simulink model "equivalent"  (R2018a)
settings: Solver=VariableStepAuto  StartTime=0.0  StopTime=10.0  RelTol=1e-3
undefined symbols (not defined in the file): DiscIntNeverNeededParam, sigbuilder_block
libraries: simulink x479
(part 1 of 10)
settings Model: Creator=cyfuzz  LastModifiedBy=ishaf
settings CodeAppCC: StateflowObjectComments=on

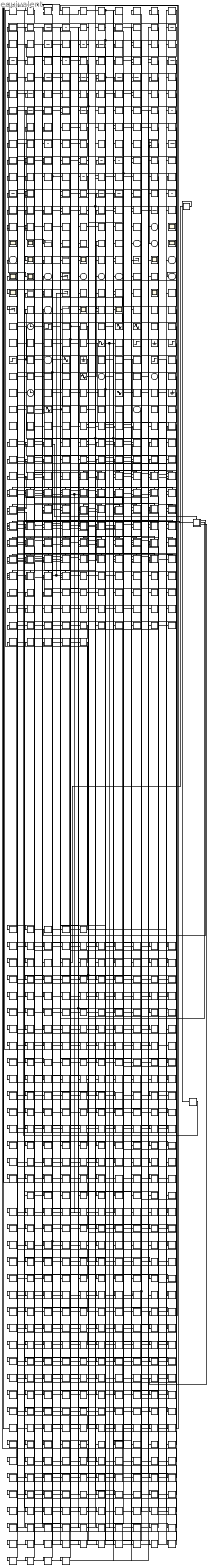
== system equivalent ==
  cfblk213 : Inport
  cfblk226 : Inport  Port=2
  cfblk229 : Inport  Port=3
  cfblk248 : Inport  Port=4
  cfblk{1,12,36,61,86,91,101,108,110,138} (10 alike) : simulink/Discrete/Transfer Fcn First Order  PoleZ=0.95  ICPrevOutput=0.0  DoSatur=off
      settings: SourceProductName=Simulink
  cfblk{10..11,16,21,37,63,66,76,80,123} (10 alike) : simulink/Continuous/PID Controller  Controller=PID  TimeDomain=Discrete-time  SampleTime=1  IntegratorMethod=Forward Euler  FilterMethod=Forward Euler  Form=Parallel  UseFilter=on  ControllerParametersSource=internal  P=1  I=1  D=0  N=100  InitialConditionSource=internal  InitialConditionForIntegrator=0  InitialConditionForFilter=0  ExternalReset=none  LimitOutput=off  UpperSaturationLimit=inf  LowerSaturationLimit=-inf  LinearizeAsGain=off  AntiWindupMode=none  Kb=1  TrackingMode=off  Kt=1  PParamMin=[]  PParamMax=[]  IParamMin=[]  IParamMax=[]  DParamMin=[]  DParamMax=[]  NParamMin=[]  NParamMax=[]  KbParamMin=[]  KbParamMax=[]  KtParamMin=[]  KtParamMax=[]  POutMin=[]  POutMax=[]  IOutMin=[]  IOutMax=[]  DOutMin=[]  DOutMax=[]  NOutMin=[]  NOutMax=[]  KbOutMin=[]  KbOutMax=[]  KtOutMin=[]  KtOutMax=[]  IntegratorOutMin=[]  IntegratorOutMax=[]  FilterOutMin=[]  FilterOutMax=[]  SumOutMin=[]  SumOutMax=[]  SumI1OutMin=[]  SumI1OutMax=[]  SumI2OutMin=[]  SumI2OutMax=[]  SumI3OutMin=[]  SumI3OutMax=[]  SumDOutMin=[]  SumDOutMax=[]  SaturationOutMin=[]  SaturationOutMax=[]  IntegratorContinuousStateAttributes=''  IntegratorStateMustResolveToSignalObject=off  IntegratorRTWStateStorageClass=Auto  FilterContinuousStateAttributes=''  FilterStateMustResolveToSignalObject=off  FilterRTWStateStorageClass=Auto  DifferentiatorICPrevScaledInput=0  DifferentiatorOutMin=[]  DifferentiatorOutMax=[]  FilterDiffOutCoefMin=[]  FilterDiffOutCoefMax=[]  SumDenOutMin=[]  SumDenOutMax=[]  SumNumOutMin=[]  SumNumOutMax=[]  ReciprocalOutMin=[]  ReciprocalOutMax=[]  DivideOutMin=[]  DivideOutMax=[]  TunerSelectOption=Transfer Function Based (PID Tuner App)
  cfblk{19,32,55,67,82,99..100,102,104,134} (10 alike) : simulink/Discrete/Difference  ICPrevInput=0.0  OutMin=[]  OutMax=[]  OutDataTypeStr=Inherit: Inherit via back propagation  OutDataType=fixdt(1, 16)  OutScaling=2^-10  DoSatur=off
  cfblk{33,42,49,57,103,121..122,126,135,345..384} (49 alike) : Delay  SampleTime=1
  cfblk{20,25,31,96,105,111} (6 alike) : DiscreteIntegrator  ICPrevOutput=DiscIntNeverNeededParam  ICPrevScaledInput=DiscIntNeverNeededParam
  cfblk{28,46,51,58,89,98,106,128} (8 alike) : simulink/Continuous/PID Controller (2DOF)  Controller=PID  TimeDomain=Discrete-time  SampleTime=1  IntegratorMethod=Forward Euler  FilterMethod=Forward Euler  Form=Parallel  UseFilter=on  ControllerParametersSource=internal  P=1  I=1  D=0  N=100  b=1  c=1  InitialConditionSource=internal  InitialConditionForIntegrator=0  InitialConditionForFilter=0  ExternalReset=none  LimitOutput=off  UpperSaturationLimit=inf  LowerSaturationLimit=-inf  LinearizeAsGain=off  AntiWindupMode=none  Kb=1  TrackingMode=off  Kt=1  PParamMin=[]  PParamMax=[]  IParamMin=[]  IParamMax=[]  DParamMin=[]  DParamMax=[]  NParamMin=[]  NParamMax=[]  bParamMin=[]  bParamMax=[]  cParamMin=[]  cParamMax=[]  KbParamMin=[]  KbParamMax=[]  KtParamMin=[]  KtParamMax=[]  POutMin=[]  POutMax=[]  IOutMin=[]  IOutMax=[]  DOutMin=[]  DOutMax=[]  NOutMin=[]  NOutMax=[]  bOutMin=[]  bOutMax=[]  cOutMin=[]  cOutMax=[]  KbOutMin=[]  KbOutMax=[]  KtOutMin=[]  KtOutMax=[]  IntegratorOutMin=[]  IntegratorOutMax=[]  FilterOutMin=[]  FilterOutMax=[]  SumOutMin=[]  SumOutMax=[]  Sum1OutMin=[]  Sum1OutMax=[]  Sum2OutMin=[]  Sum2OutMax=[]  Sum3OutMin=[]  Sum3OutMax=[]  SumI1OutMin=[]  SumI1OutMax=[]  SumI2OutMin=[]  SumI2OutMax=[]  SumI3OutMin=[]  SumI3OutMax=[]  SumDOutMin=[]  SumDOutMax=[]  SaturationOutMin=[]  SaturationOutMax=[]  IntegratorContinuousStateAttributes=''  IntegratorStateMustResolveToSignalObject=off  IntegratorRTWStateStorageClass=Auto  FilterContinuousStateAttributes=''  FilterStateMustResolveToSignalObject=off  FilterRTWStateStorageClass=Auto  DifferentiatorICPrevScaledInput=0  DifferentiatorOutMin=[]  DifferentiatorOutMax=[]  FilterDiffOutCoefMin=[]  FilterDiffOutCoefMax=[]  SumDenOutMin=[]  SumDenOutMax=[]  SumNumOutMin=[]  SumNumOutMax=[]  ReciprocalOutMin=[]  ReciprocalOutMax=[]  DivideOutMin=[]  DivideOutMax=[]  TunerSelectOption=Transfer Function Based (PID Tuner App)
  cfblk{35,53,87,94,107,119,125,133} (8 alike) : simulink/Discrete/Transfer Fcn Real Zero  ZeroZ=0.75  ICPrevInput=0.0  DoSatur=off
      settings: SourceProductName=Simulink  SourceProductBaseCode=SL
  cfblk{18,24,54,56,69,71,75,85,109,130} (10 alike) : simulink/Discrete/Transfer Fcn Lead or Lag  PoleZ=0.95  ZeroZ=0.75  ICPrevOutput=0.0  ICPrevInput=0.0  DoSatur=off
      settings: SourceProductName=Simulink  SourceProductBaseCode=SL
  cfblk{64,92,112,131..132} (5 alike) : Delay  DelayLengthSource=Input port  SampleTime=1
      settings: InputPortMap=u0,p1
  cfblk{7,15,22,27,30,41,44,60,81,113} (10 alike) : DiscreteZeroPole  Poles=[0 0.5]  Gain=1
  cfblk{3,38..39,77,93,95,114,124,127} (9 alike) : Delay  ShowEnablePort=on  SampleTime=1
      settings: InputPortMap=u0,e6
  cfblk{17,50,72,78..79,115} (6 alike) : simulink/Discrete/Tapped Delay  vinit=0.0  samptime=-1  NumDelays=1  DelayOrder=Oldest  includeCurrent=off
  cfblk{23,45,116..117} (4 alike) : DiscreteTransferFcn  SampleTime=1
  cfblk{2,4..6,59,68,73..74,118,137} (10 alike) : DiscreteFir  SampleTime=1
  cfblk{14,29,34,70,83,97,120} (7 alike) : UnitDelay
  cfblk{13,26,40,43,47..48,52,62,65,90,129} (11 alike) : DiscreteFilter  SampleTime=1
  cfblk{8..9,84,88,136} (5 alike) : DiscreteStateSpace
  cfblk{140..142,150,152,155,159,161..162,171,179,185,187} (13 alike) : Scope
      cfblk140 settings: Floating=on
      cfblk141 settings: Floating=on
      cfblk142 settings: Floating=on
      cfblk150 settings: Floating=on
      cfblk179 settings: Floating=on
  cfblk{143,154,172,184} (4 alike) : Display
  cfblk144 : ToWorkspace  VariableName=lgebsck  SaveFormat=Timeseries  SampleTime=-1
  cfblk145 : ToWorkspace  VariableName=bihdjlv  SaveFormat=Timeseries  SampleTime=-1
  cfblk{146,157,173,177,186} (5 alike) : simulink/Sinks/XY Graph  xmin=-1  xmax=1  ymin=-1  ymax=1  st=-1
  cfblk147 : ToWorkspace  VariableName=xeqpvpt  SaveFormat=Timeseries  SampleTime=-1
  cfblk153 : ToFile  Filename=ktyo  SaveFormat=Timeseries
  cfblk156 : ToFile  Filename=grzb  SaveFormat=Timeseries
  cfblk{158,164,174,181} (4 alike) : Terminator
  cfblk168 : ToWorkspace  VariableName=rlyvhgw  SaveFormat=Timeseries  SampleTime=-1
  cfblk169 : ToFile  Filename=ghct  SaveFormat=Timeseries
  cfblk175 : ToFile  Filename=zzva  SaveFormat=Timeseries
  cfblk176 : ToWorkspace  VariableName=iqauudf  SaveFormat=Timeseries  SampleTime=-1
  cfblk178 : ToFile  Filename=xfod  SaveFormat=Timeseries
  cfblk180 : ToWorkspace  VariableName=neyrlfn  SaveFormat=Timeseries  SampleTime=-1
  cfblk182 : ToFile  Filename=fvos  SaveFormat=Timeseries
  cfblk188 : ToWorkspace  VariableName=xtilwmv  SaveFormat=Timeseries  SampleTime=-1
  cfblk{189,203,231,247,250..251} (6 alike) : simulink/Sources/Repeating Sequence Interpolated  OutValues=[3 1 4 2 1].'  TimeValues=[0 0.1 0.5 0.6 1].'  LookUpMeth=Interpolation-Use End Values  tsamp=0.01  OutMin=[]  OutMax=[]  OutDataTypeStr=double  OutputDataTypeScalingMode=double  OutDataType=fixdt(0,8)  OutScaling=2^-10
  cfblk190 : simulink/Sources/Repeating Sequence  rep_seq_t=[0 2]  rep_seq_y=[0 2]
  cfblk191 : simulink/Sources/Repeating Sequence  rep_seq_t=[0 2]  rep_seq_y=[0 2]
  cfblk192 : Clock
  cfblk193 : Step  After=18  SampleTime=0
  cfblk194 : SignalGenerator  Units=rad/sec
  cfblk{195,216,234,236,238..239} (6 alike) : simulink/Sources/Chirp Signal  f1=0.1  T=100  f2=1
  cfblk196 : Constant  Value=8987
  cfblk{197..198,206,214,225,237,243} (7 alike) : Sin  SampleTime=0
  cfblk{199,230,235,241} (4 alike) : RandomNumber  SampleTime=0.1
  cfblk200 : simulink/Sources/Counter Free-Running  NumBits=16  tsamp=-1
  cfblk{201,212,220,249} (4 alike) : simulink/Sources/Band-Limited White Noise  Cov=[0.1]  Ts=0.1  seed=[23341]
  cfblk202 : UniformRandomNumber  SampleTime=0.1
  cfblk204 : Subsystem  Tag=STV Subsys  LoadFcn=sigbuilder_block('load');  StartFcn=sigbuilder_block('start');  StopFcn=sigbuilder_block('stop');  ClipboardFcn=sigbuilder_block('clipboard');  mask(Sigbuilder block){tuvar=[0:10]}
      mask help: Simulink:masks:SigbuilderBlock_MD
      mask init:
      | if ~strcmp(get_param(bdroot(gcbh),'SimulationStatus'),'stopped') tuvar = sigbuilder_block('maskInit'); end
      settings: CopyFcn=sigbuilder_block('copy');  DeleteFcn=sigbuilder_block('delete');  ModelCloseFcn=sigbuilder_block('modelClose');  PreSaveFcn=sigbuilder_block('preSave');  PauseFcn=sigbuilder_block('pause');  ContinueFcn=sigbuilder_block('continue');  NameChangeFcn=sigbuilder_block('namechange');  OpenFcn=sigbuilder_block('open',[437.6 199.2 550.4 400 ]);  CloseFcn=sigbuilder_block('close');
      mask Display: plot(0, 0, 100, 100,[2, 2, 32, 32, 2], [68, 8, 8, 68, 68],[32, 2], [38, 38], [32, 19, 2],[53, 60, 44], [32, 17, 17, 2],[16, 16, 31, 31]);txt = getActiveGroup(gcbh);text(2, 100, txt,'verticalAlignment', 'top');
  cfblk205 : DiscretePulseGenerator  PulseType=Time based  Period=10  PulseWidth=5
  cfblk207 : simulink/Sources/Repeating Sequence  rep_seq_t=[0 2]  rep_seq_y=[0 2]
  cfblk208 : Step  After=83  SampleTime=0
  cfblk209 : Ground
  cfblk210 : Step  After=27  SampleTime=0
  cfblk211 : Step  After=11  SampleTime=0
  cfblk215 : Ground
  cfblk{217,222,253..254} (4 alike) : simulink/Sources/Repeating Sequence Stair  OutValues=[3 1 4 2 1].'  tsamp=-1  OutMin=[]  OutMax=[]  OutDataTypeStr=double  OutputDataTypeScalingMode=double  OutDataType=fixdt(0,8)  ConRadixGroup=Best Precision: Vector-wise  OutScaling=2^-12
  cfblk218 : Constant  Value=1094
  cfblk219 : Step  After=49  SampleTime=0
  cfblk221 : DigitalClock
  cfblk223 : simulink/Sources/Ramp  slope=1  start=0  InitialOutput=0
  cfblk224 : Constant  Value=9975
  cfblk227 : simulink/Sources/Counter Limited  uplimit=7  tsamp=-1
  cfblk228 : Subsystem  Tag=STV Subsys  LoadFcn=sigbuilder_block('load');  StartFcn=sigbuilder_block('start');  StopFcn=sigbuilder_block('stop');  ClipboardFcn=sigbuilder_block('clipboard');  mask(Sigbuilder block){tuvar=[0:10]}
      mask help: Simulink:masks:SigbuilderBlock_MD
      mask init:
      | if ~strcmp(get_param(bdroot(gcbh),'SimulationStatus'),'stopped') tuvar = sigbuilder_block('maskInit'); end
      settings: CopyFcn=sigbuilder_block('copy');  DeleteFcn=sigbuilder_block('delete');  ModelCloseFcn=sigbuilder_block('modelClose');  PreSaveFcn=sigbuilder_block('preSave');  PauseFcn=sigbuilder_block('pause');  ContinueFcn=sigbuilder_block('continue');  NameChangeFcn=sigbuilder_block('namechange');  OpenFcn=sigbuilder_block('open',[437.6 199.2 550.4 400 ]);  CloseFcn=sigbuilder_block('close');
      mask Display: plot(0, 0, 100, 100,[2, 2, 32, 32, 2], [68, 8, 8, 68, 68],[32, 2], [38, 38], [32, 19, 2],[53, 60, 44], [32, 17, 17, 2],[16, 16, 31, 31]);txt = getActiveGroup(gcbh);text(2, 100, txt,'verticalAlignment', 'top');
  cfblk232 : Clock
  cfblk233 : SignalGenerator  Units=rad/sec
  cfblk240 : Ground
  cfblk242 : Subsystem  Tag=STV Subsys  LoadFcn=sigbuilder_block('load');  StartFcn=sigbuilder_block('start');  StopFcn=sigbuilder_block('stop');  ClipboardFcn=sigbuilder_block('clipboard');  mask(Sigbuilder block){tuvar=[0:10]}
      mask help: Simulink:masks:SigbuilderBlock_MD
      mask init:
      | if ~strcmp(get_param(bdroot(gcbh),'SimulationStatus'),'stopped') tuvar = sigbuilder_block('maskInit'); end
      settings: CopyFcn=sigbuilder_block('copy');  DeleteFcn=sigbuilder_block('delete');  ModelCloseFcn=sigbuilder_block('modelClose');  PreSaveFcn=sigbuilder_block('preSave');  PauseFcn=sigbuilder_block('pause');  ContinueFcn=sigbuilder_block('continue');  NameChangeFcn=sigbuilder_block('namechange');  OpenFcn=sigbuilder_block('open',[437.6 199.2 550.4 400 ]);  CloseFcn=sigbuilder_block('close');
      mask Display: plot(0, 0, 100, 100,[2, 2, 32, 32, 2], [68, 8, 8, 68, 68],[32, 2], [38, 38], [32, 19, 2],[53, 60, 44], [32, 17, 17, 2],[16, 16, 31, 31]);txt = getActiveGroup(gcbh);text(2, 100, txt,'verticalAlignment', 'top');
  cfblk244 : simulink/Sources/Counter Limited  uplimit=7  tsamp=-1
  cfblk245 : SignalGenerator  Units=rad/sec
  cfblk246 : DigitalClock
  cfblk252 : DigitalClock
  cfblk{255..284} (30 alike) : If  SampleTime=1
  cfblk285 : Subsystem  TreatAsAtomicUnit=on
  cfblk286 : Subsystem  TreatAsAtomicUnit=on
  cfblk287 : Subsystem  TreatAsAtomicUnit=on
  cfblk288 : Subsystem  TreatAsAtomicUnit=on
  cfblk289 : Subsystem  TreatAsAtomicUnit=on
  cfblk290 : Subsystem  TreatAsAtomicUnit=on
  cfblk291 : Subsystem  TreatAsAtomicUnit=on
  cfblk292 : Subsystem  TreatAsAtomicUnit=on
  cfblk293 : Subsystem  TreatAsAtomicUnit=on
  cfblk294 : Subsystem  TreatAsAtomicUnit=on
  cfblk295 : Subsystem  TreatAsAtomicUnit=on
  cfblk296 : Subsystem  TreatAsAtomicUnit=on
  cfblk297 : Subsystem  TreatAsAtomicUnit=on
  cfblk298 : Subsystem  TreatAsAtomicUnit=on
  cfblk299 : Subsystem  TreatAsAtomicUnit=on
  cfblk300 : Subsystem  TreatAsAtomicUnit=on
  cfblk301 : Subsystem  TreatAsAtomicUnit=on
  cfblk302 : Subsystem  TreatAsAtomicUnit=on
  cfblk303 : Subsystem  TreatAsAtomicUnit=on
  cfblk304 : Subsystem  TreatAsAtomicUnit=on
  cfblk305 : Subsystem  TreatAsAtomicUnit=on
  cfblk306 : Subsystem  TreatAsAtomicUnit=on
  cfblk307 : Subsystem  TreatAsAtomicUnit=on
  cfblk308 : Subsystem  TreatAsAtomicUnit=on
  cfblk309 : Subsystem  TreatAsAtomicUnit=on
  cfblk310 : Subsystem  TreatAsAtomicUnit=on
  cfblk311 : Subsystem  TreatAsAtomicUnit=on
  cfblk312 : Subsystem  TreatAsAtomicUnit=on
  cfblk313 : Subsystem  TreatAsAtomicUnit=on
  cfblk314 : Subsystem  TreatAsAtomicUnit=on
  cfblk315 : Subsystem  TreatAsAtomicUnit=on
  cfblk316 : Subsystem  TreatAsAtomicUnit=on
  cfblk317 : Subsystem  TreatAsAtomicUnit=on
  cfblk318 : Subsystem  TreatAsAtomicUnit=on
  cfblk319 : Subsystem  TreatAsAtomicUnit=on
  cfblk320 : Subsystem  TreatAsAtomicUnit=on
  cfblk321 : Subsystem  TreatAsAtomicUnit=on
  cfblk322 : Subsystem  TreatAsAtomicUnit=on
  cfblk323 : Subsystem  TreatAsAtomicUnit=on
  cfblk324 : Subsystem  TreatAsAtomicUnit=on
  cfblk325 : Subsystem  TreatAsAtomicUnit=on
  cfblk326 : Subsystem  TreatAsAtomicUnit=on
  cfblk327 : Subsystem  TreatAsAtomicUnit=on
  cfblk328 : Subsystem  TreatAsAtomicUnit=on
  cfblk329 : Subsystem  TreatAsAtomicUnit=on
  cfblk330 : Subsystem  TreatAsAtomicUnit=on
  cfblk331 : Subsystem  TreatAsAtomicUnit=on
  cfblk332 : Subsystem  TreatAsAtomicUnit=on
  cfblk333 : Subsystem  TreatAsAtomicUnit=on
  cfblk334 : Subsystem  TreatAsAtomicUnit=on
  cfblk335 : Subsystem  TreatAsAtomicUnit=on
  cfblk336 : Subsystem  TreatAsAtomicUnit=on
  cfblk337 : Subsystem  TreatAsAtomicUnit=on
  cfblk338 : Subsystem  TreatAsAtomicUnit=on
  cfblk339 : Subsystem  TreatAsAtomicUnit=on
  cfblk340 : Subsystem  TreatAsAtomicUnit=on
  cfblk341 : Subsystem  TreatAsAtomicUnit=on
  cfblk342 : Subsystem  TreatAsAtomicUnit=on
  cfblk343 : Subsystem  TreatAsAtomicUnit=on
  cfblk344 : Subsystem  TreatAsAtomicUnit=on
  cfblk385 : DataTypeConversion  OutDataTypeStr=double
  cyemi_{0..42,44..47,49..57,59..77,79..113,124,165..166,202..203,210..211,215..218,228..229,234..236,304..306,349..351,361..362,372..373,447..448,450..451,457..459,498..502,517..518,557,595..596,634..635,663..667,705,723..728,739..740,773..774,789..791,805..808,816..817,827..828,889,929..932,955..956,963,970..971,987..988,1002..1004,1061..1062,1088..1089,1103..1104,1155..1157,1230..1231,1236..1240,1246..1247,1282..1284,1291..1292,1302..1303,1376..1377,1414..1415,1423..1424,1448..1449,1470,1538,1546..1548,1560..1562,1567..1568,1604..1605,1639..1641,1683,1692,1708..1710,1747..1791,1793..1859,1861..1870} (372 alike) : DataTypeConversion  OutDataTypeStr=double
  cyemi_1792 : DataTypeConversion  OutDataTypeStr=uint16
  cyemi_{43,48,237,1860} (4 alike) : DataTypeConversion  OutDataTypeStr=uint32
  cyemi_58 : DataTypeConversion  OutDataTypeStr=uint8
  cyemi_78 : DataTypeConversion  OutDataTypeStr=uint8
  cfblk139 : Outport
  cfblk148 : Outport  Port=2
  cfblk149 : Outport  Port=3
  cfblk151 : Outport  Port=4
  cfblk160 : Outport  Port=5
  cfblk163 : Outport  Port=6
  cfblk165 : Outport  Port=7
  cfblk166 : Outport  Port=8
  cfblk167 : Outport  Port=9
  cfblk170 : Outport  Port=10
  cfblk183 : Outport  Port=11
  wires:
  cfblk79/1 -> cfblk149/1
  cfblk61/1 -> cfblk143/1
  cfblk2/1 -> cfblk162/1
  cfblk10/1 -> cfblk148/1
  cfblk225/1 -> cfblk146/1
  cfblk323/1(cfblk2) -> cfblk183/1
  cfblk46/1 -> cyemi_457/1, cyemi_1568/1
  cfblk197/1 -> cfblk172/1
  cfblk7/1 -> cfblk181/1
  cfblk307/1(cfblk2) -> cfblk166/1
  cfblk243/1 -> cyemi_727/1, cyemi_1846/1, cfblk177/2
  cfblk20/1 -> cyemi_110/1, cyemi_1548/1
  cfblk194/1 -> cyemi_38/1, cyemi_740/1
  cfblk206/1 -> cyemi_667/1, cyemi_1853/1
  cfblk217/1 -> cyemi_1088/1, cyemi_1239/1
  cfblk8/1 -> cfblk186/1
  cfblk69/1 -> cyemi_29/1, cyemi_236/1
  cfblk211/1 -> cfblk146/2, cyemi_666/1
  cfblk214/1 -> cyemi_234/1, cyemi_1867/1
  cfblk314/2(cfblk8) -> cfblk160/1
  cfblk80/1 -> cfblk170/1
  cfblk118/1 -> cfblk186/2, cyemi_1778/1
  cfblk290/1(cfblk2) -> cfblk151/1
  cfblk231/1 -> cyemi_22/1, cyemi_932/1
  cfblk98/1 -> cyemi_235/1, cyemi_1753/1
  cfblk195/1 -> cyemi_1869/1, cyemi_1870/1
  cfblk301/1(cfblk2) -> cfblk139/1
  cfblk38/1 -> cyemi_1284/1, cyemi_1424/1
  cfblk298/2(cfblk9) -> cfblk159/1, cyemi_106/1
  cfblk343/1(cfblk2) -> cfblk174/1, cyemi_82/1
  cfblk310/4(cfblk16) -> cfblk161/1
  cfblk29/1 -> cfblk152/1
  cfblk330/2(cfblk13) -> cfblk165/1
  cfblk125/1 -> cfblk155/1
  cfblk335/2(cfblk11) -> cfblk157/1
  cfblk312/1(cfblk2) -> cyemi_725/1, cyemi_1758/1
  cfblk331/3(cfblk11) -> cfblk154/1
  cfblk103/1 -> cyemi_728/1, cyemi_1777/1
  cfblk57/1 -> cfblk158/1
  cfblk301/2(cfblk13) -> cfblk187/1
  cfblk34/1 -> cyemi_54/1, cyemi_1710/1
  cfblk81/1 -> cfblk157/2
  cfblk331/4(cfblk12) -> cfblk184/1
  cfblk21/1 -> cfblk167/1
  cfblk16/1 -> cyemi_889/1, cyemi_1546/1
  cfblk229/1 -> cyemi_237/1, cyemi_1860/1
  cfblk304/1(cfblk2) -> cfblk173/1
  cfblk18/1 -> cfblk164/1
  cfblk25/1 -> cfblk185/1
  cfblk294/2(cfblk14) -> cyemi_21/1, cyemi_726/1
  cfblk60/1 -> cyemi_1240/1, cyemi_1811/1
  cfblk295/2(cfblk11) -> cfblk173/2
  cfblk134/1 -> cfblk171/1
  cfblk6/1 -> cyemi_10/1, cyemi_963/1
  cfblk320/4(cfblk15) -> cfblk163/1
  cfblk106/1 -> cfblk177/1
  cfblk255/1 -> cfblk285/Action
  cfblk255/2 -> cfblk286/Action
  cfblk256/1 -> cfblk287/Action
  cfblk256/2 -> cfblk288/Action
  cfblk257/1 -> cfblk289/Action
  cfblk257/2 -> cfblk290/Action
  cfblk258/1 -> cfblk291/Action
  cfblk258/2 -> cfblk292/Action
  cfblk259/1 -> cfblk293/Action
  cfblk259/2 -> cfblk294/Action
  cfblk260/1 -> cfblk295/Action
  cfblk260/2 -> cfblk296/Action
  cfblk261/1 -> cfblk297/Action
  cfblk261/2 -> cfblk298/Action
  cfblk262/1 -> cfblk299/Action
  cfblk262/2 -> cfblk300/Action
  cfblk263/1 -> cfblk301/Action
  cfblk263/2 -> cfblk302/Action
  cfblk264/1 -> cfblk303/Action
  cfblk264/2 -> cfblk304/Action
  cfblk265/1 -> cfblk305/Action
  cfblk265/2 -> cfblk306/Action
  cfblk266/1 -> cfblk307/Action
  cfblk266/2 -> cfblk308/Action
  cfblk267/1 -> cfblk309/Action
  cfblk267/2 -> cfblk310/Action
  cfblk268/1 -> cfblk311/Action
  cfblk268/2 -> cfblk312/Action
  cfblk269/1 -> cfblk313/Action
  cfblk269/2 -> cfblk314/Action
  cfblk270/1 -> cfblk315/Action
  cfblk270/2 -> cfblk316/Action
  cfblk271/1 -> cfblk317/Action
  cfblk271/2 -> cfblk318/Action
  cfblk272/1 -> cfblk319/Action
  cfblk272/2 -> cfblk320/Action
  cfblk273/1 -> cfblk321/Action
  cfblk273/2 -> cfblk322/Action
  cfblk274/1 -> cfblk323/Action
  cfblk274/2 -> cfblk324/Action
  cfblk275/1 -> cfblk325/Action
  cfblk275/2 -> cfblk326/Action
  cfblk276/1 -> cfblk327/Action
  cfblk276/2 -> cfblk328/Action
  cfblk277/1 -> cfblk329/Action
  cfblk277/2 -> cfblk330/Action
  cfblk278/1 -> cfblk331/Action
  cfblk278/2 -> cfblk332/Action
  cfblk279/1 -> cfblk333/Action
  cfblk279/2 -> cfblk334/Action
  cfblk280/1 -> cfblk335/Action
  cfblk280/2 -> cfblk336/Action
  cfblk281/1 -> cfblk337/Action
  cfblk281/2 -> cfblk338/Action
  cfblk282/1 -> cfblk339/Action
  cfblk282/2 -> cfblk340/Action
  cfblk283/1 -> cfblk341/Action
  cfblk283/2 -> cfblk342/Action
  cfblk284/1 -> cfblk343/Action
  cfblk284/2 -> cfblk344/Action
  cyemi_0/1 -> cfblk1/1
  cfblk362/1 -> cyemi_0/1
  cyemi_1/1 -> cfblk10/1
  cfblk315/4(cfblk13) -> cyemi_1/1
  cyemi_2/1 -> cfblk100/1
  cfblk302/1(cfblk2) -> cyemi_2/1
  cyemi_3/1 -> cfblk101/1
  cfblk286/1(cfblk2) -> cyemi_3/1
  cyemi_4/1 -> cfblk102/1
  cfblk293/2(cfblk12) -> cyemi_4/1
  cyemi_5/1 -> cfblk103/1
  cfblk314/1(cfblk2) -> cyemi_5/1
  cyemi_6/1 -> cfblk104/1
  cfblk230/1 -> cyemi_6/1
  cyemi_7/1 -> cfblk105/1
  cfblk296/1(cfblk2) -> cyemi_7/1
  cyemi_8/1 -> cfblk106/1
  cfblk224/1 -> cyemi_8/1
  cyemi_9/1 -> cfblk106/2
  cfblk338/2(cfblk8) -> cyemi_9/1
  cyemi_10/1 -> cfblk107/1
  cyemi_11/1 -> cfblk108/1
  cfblk47/1 -> cyemi_11/1
  cyemi_12/1 -> cfblk109/1
  cfblk205/1 -> cyemi_12/1
  cyemi_13/1 -> cfblk11/1
  cfblk122/1 -> cyemi_13/1
  cyemi_14/1 -> cfblk110/1
  cfblk56/1 -> cyemi_14/1
  cyemi_15/1 -> cfblk111/1
  cfblk327/1(cfblk2) -> cyemi_15/1
  cyemi_16/1 -> cfblk112/1
  cfblk108/1 -> cyemi_16/1
  cyemi_17/1 -> cfblk112/2
  cfblk201/1 -> cyemi_17/1
  cyemi_18/1 -> cfblk113/1
  cfblk385/1 -> cyemi_18/1
  cyemi_19/1 -> cfblk114/1
  cfblk221/1 -> cyemi_19/1
  cyemi_20/1 -> cfblk114/2
  cfblk213/1 -> cyemi_20/1
  cyemi_21/1 -> cfblk115/1
  cyemi_22/1 -> cfblk116/1
  cyemi_23/1 -> cfblk117/1
  cfblk107/1 -> cyemi_23/1
  cyemi_24/1 -> cfblk118/1
  cfblk334/1(cfblk2) -> cyemi_24/1
  cyemi_25/1 -> cfblk119/1
  cfblk331/1(cfblk2) -> cyemi_25/1
  cyemi_26/1 -> cfblk12/1
  cfblk320/1(cfblk2) -> cyemi_26/1
  cyemi_27/1 -> cfblk120/1
  cfblk291/1(cfblk2) -> cyemi_27/1
  cyemi_28/1 -> cfblk121/1
  cfblk316/1(cfblk2) -> cyemi_28/1
  cyemi_29/1 -> cfblk122/1
  cyemi_30/1 -> cfblk123/1
  cfblk136/1 -> cyemi_30/1
  cyemi_31/1 -> cfblk124/1
  cfblk70/1 -> cyemi_31/1
  cyemi_32/1 -> cfblk124/2
  cfblk333/1(cfblk2) -> cyemi_32/1
  cyemi_33/1 -> cfblk125/1
  cfblk252/1 -> cyemi_33/1
  cyemi_34/1 -> cfblk126/1
  cfblk239/1 -> cyemi_34/1
  cyemi_35/1 -> cfblk127/1
  cfblk382/1 -> cyemi_35/1
  cyemi_36/1 -> cfblk127/2
  cfblk83/1 -> cyemi_36/1
  cyemi_37/1 -> cfblk128/1
  cfblk299/3(cfblk15) -> cyemi_37/1
  cyemi_38/1 -> cfblk128/2
  cyemi_39/1 -> cfblk129/1
  cfblk9/1 -> cyemi_39/1
  cyemi_40/1 -> cfblk13/1
  cfblk189/1 -> cyemi_40/1
  cyemi_41/1 -> cfblk130/1
  cfblk314/3(cfblk9) -> cyemi_41/1
  cyemi_42/1 -> cfblk131/1
  cfblk287/1(cfblk2) -> cyemi_42/1
  cyemi_43/1 -> cfblk131/2
  cfblk135/1 -> cyemi_43/1
  cyemi_44/1 -> cfblk132/1
  cfblk367/1 -> cyemi_44/1
  cyemi_45/1 -> cfblk132/2
  cfblk304/3(cfblk9) -> cyemi_45/1
  cyemi_46/1 -> cfblk133/1
  cfblk44/1 -> cyemi_46/1
  cyemi_47/1 -> cfblk134/1
  cfblk286/2(cfblk10) -> cyemi_47/1
  cyemi_48/1 -> cfblk135/1
  cfblk302/2(cfblk13) -> cyemi_48/1
  cyemi_49/1 -> cfblk136/1
  cfblk28/1 -> cyemi_49/1
  cyemi_50/1 -> cfblk137/1
  cfblk305/1(cfblk2) -> cyemi_50/1
  cyemi_51/1 -> cfblk138/1
  cfblk67/1 -> cyemi_51/1
  cyemi_52/1 -> cfblk14/1
  cfblk84/1 -> cyemi_52/1
  cyemi_53/1 -> cfblk144/1
  cfblk325/2(cfblk7) -> cyemi_53/1
  cyemi_54/1 -> cfblk145/1
  cyemi_55/1 -> cfblk147/1
  cfblk328/2(cfblk9) -> cyemi_55/1
  cyemi_56/1 -> cfblk15/1
  cfblk112/1 -> cyemi_56/1
  cyemi_57/1 -> cfblk153/1
  cfblk326/2(cfblk10) -> cyemi_57/1
  cyemi_58/1 -> cfblk156/1
  cfblk244/1 -> cyemi_58/1
  cyemi_59/1 -> cfblk16/1
  cfblk242/1(Signal 1) -> cyemi_59/1
  cyemi_60/1 -> cfblk168/1
  cfblk330/3(cfblk14) -> cyemi_60/1
  cyemi_61/1 -> cfblk169/1
  cfblk303/1(cfblk2) -> cyemi_61/1
  cyemi_62/1 -> cfblk17/1
  cfblk316/3(cfblk11) -> cyemi_62/1
  cyemi_63/1 -> cfblk175/1
  cfblk92/1 -> cyemi_63/1
  cyemi_64/1 -> cfblk176/1
  cfblk289/2(cfblk7) -> cyemi_64/1
  cyemi_65/1 -> cfblk178/1
  cfblk137/1 -> cyemi_65/1
  cyemi_66/1 -> cfblk18/1
  cfblk119/1 -> cyemi_66/1
  cyemi_67/1 -> cfblk180/1
  cfblk104/1 -> cyemi_67/1
  cyemi_68/1 -> cfblk182/1
  cfblk85/1 -> cyemi_68/1
  cyemi_69/1 -> cfblk188/1
  cfblk138/1 -> cyemi_69/1
  cyemi_70/1 -> cfblk19/1
  cfblk121/1 -> cyemi_70/1
  cyemi_71/1 -> cfblk2/1
  cfblk323/2(cfblk17) -> cyemi_71/1
  cyemi_72/1 -> cfblk20/1
  cfblk199/1 -> cyemi_72/1
  cyemi_73/1 -> cfblk21/1
  cfblk74/1 -> cyemi_73/1
  cyemi_74/1 -> cfblk22/1
  cfblk222/1 -> cyemi_74/1
  cyemi_75/1 -> cfblk23/1
  cfblk55/1 -> cyemi_75/1
  cyemi_76/1 -> cfblk24/1
  cfblk308/1(cfblk2) -> cyemi_76/1
  cyemi_77/1 -> cfblk25/1
  cfblk51/1 -> cyemi_77/1
  cyemi_78/1 -> cfblk255/1
  cfblk227/1 -> cyemi_78/1
  cyemi_79/1 -> cfblk256/1
  cfblk310/2(cfblk14) -> cyemi_79/1
  cyemi_80/1 -> cfblk257/1
  cfblk384/1 -> cyemi_80/1
  cyemi_81/1 -> cfblk258/1
  cfblk226/1 -> cyemi_81/1
  cyemi_82/1 -> cfblk259/1
  cyemi_83/1 -> cfblk26/1
  cfblk228/1(Signal 1) -> cyemi_83/1
  cyemi_84/1 -> cfblk260/1
  cfblk68/1 -> cyemi_84/1
  cyemi_85/1 -> cfblk261/1
  cfblk251/1 -> cyemi_85/1
  cyemi_86/1 -> cfblk262/1
  cfblk296/3(cfblk13) -> cyemi_86/1
  cyemi_87/1 -> cfblk263/1
  cfblk358/1 -> cyemi_87/1
  cyemi_88/1 -> cfblk264/1
  cfblk319/1(cfblk2) -> cyemi_88/1
  cyemi_89/1 -> cfblk265/1
  cfblk249/1 -> cyemi_89/1
  cyemi_90/1 -> cfblk266/1
  cfblk332/4(cfblk12) -> cyemi_90/1
  cyemi_91/1 -> cfblk267/1
  cfblk202/1 -> cyemi_91/1
  cyemi_92/1 -> cfblk268/1
  cfblk115/1 -> cyemi_92/1
  cyemi_93/1 -> cfblk269/1
  cfblk128/1 -> cyemi_93/1
  cyemi_94/1 -> cfblk27/1
  cfblk311/1(cfblk2) -> cyemi_94/1
  cyemi_95/1 -> cfblk270/1
  cfblk240/1 -> cyemi_95/1
  cyemi_96/1 -> cfblk271/1
  cfblk82/1 -> cyemi_96/1
  cyemi_97/1 -> cfblk272/1
  cfblk191/1 -> cyemi_97/1
  cyemi_98/1 -> cfblk273/1
  cfblk348/1 -> cyemi_98/1
  cyemi_99/1 -> cfblk274/1
  cfblk15/1 -> cyemi_99/1
  cyemi_100/1 -> cfblk275/1
  cfblk130/1 -> cyemi_100/1
  cyemi_101/1 -> cfblk276/1
  cfblk131/1 -> cyemi_101/1
  cyemi_102/1 -> cfblk277/1
  cfblk190/1 -> cyemi_102/1
  cyemi_103/1 -> cfblk278/1
  cfblk340/1(cfblk2) -> cyemi_103/1
  cyemi_104/1 -> cfblk279/1
  cfblk219/1 -> cyemi_104/1
  cyemi_105/1 -> cfblk28/1
  cfblk52/1 -> cyemi_105/1
  cyemi_106/1 -> cfblk28/2
  cyemi_107/1 -> cfblk280/1
  cfblk87/1 -> cyemi_107/1
  cyemi_108/1 -> cfblk281/1
  cfblk65/1 -> cyemi_108/1
  cyemi_109/1 -> cfblk282/1
  cfblk204/1(Signal 1) -> cyemi_109/1
  cyemi_110/1 -> cfblk283/1
  cyemi_111/1 -> cfblk284/1
  cfblk48/1 -> cyemi_111/1
  cyemi_112/1 -> cfblk285/1(cfblk1)
  cfblk99/1 -> cyemi_112/1
  cyemi_113/1 -> cfblk285/2(cfblk11)
  cfblk313/3(cfblk15) -> cyemi_113/1
  cyemi_124/1 -> cfblk286/1(cfblk1)
  cfblk114/1 -> cyemi_124/1
  cyemi_165/1 -> cfblk287/1(cfblk1)
  cfblk208/1 -> cyemi_165/1
  cyemi_166/1 -> cfblk287/2(cfblk12)
  cfblk340/2(cfblk13) -> cyemi_166/1
  cyemi_202/1 -> cfblk288/1(cfblk1)
  cfblk58/1 -> cyemi_202/1
  cyemi_203/1 -> cfblk288/2(cfblk7)
  cfblk310/3(cfblk15) -> cyemi_203/1
  cyemi_210/1 -> cfblk289/1(cfblk1)
  cfblk45/1 -> cyemi_210/1
  cyemi_211/1 -> cfblk289/2(cfblk6)
  cfblk245/1 -> cyemi_211/1
  cyemi_215/1 -> cfblk29/1
  cfblk31/1 -> cyemi_215/1
  cyemi_216/1 -> cfblk290/1(cfblk1)
  cfblk378/1 -> cyemi_216/1
  cyemi_217/1 -> cfblk290/2(cfblk9)
  cfblk346/1 -> cyemi_217/1
  cyemi_218/1 -> cfblk290/3(cfblk10)
  cfblk42/1 -> cyemi_218/1
  cyemi_228/1 -> cfblk291/1(cfblk1)
  cfblk342/1(cfblk2) -> cyemi_228/1
  cyemi_229/1 -> cfblk291/2(cfblk7)
  cfblk27/1 -> cyemi_229/1
  cyemi_234/1 -> cfblk292/1(cfblk1)
  cyemi_235/1 -> cfblk292/2(cfblk13)
  cyemi_236/1 -> cfblk292/3(cfblk14)
  cyemi_237/1 -> cfblk292/4(cfblk15)
  cyemi_304/1 -> cfblk293/1(cfblk1)
  cfblk365/1 -> cyemi_304/1
  cyemi_305/1 -> cfblk293/2(cfblk10)
  cfblk359/1 -> cyemi_305/1
  cyemi_306/1 -> cfblk293/3(cfblk11)
  cfblk11/1 -> cyemi_306/1
  cyemi_349/1 -> cfblk294/1(cfblk1)
  cfblk381/1 -> cyemi_349/1
  cyemi_350/1 -> cfblk294/2(cfblk12)
  cfblk352/1 -> cyemi_350/1
  cyemi_351/1 -> cfblk294/3(cfblk13)
  cfblk301/4(cfblk15) -> cyemi_351/1
  cyemi_361/1 -> cfblk295/1(cfblk1)
  cfblk297/2(cfblk5) -> cyemi_361/1
  cyemi_362/1 -> cfblk295/2(cfblk10)
  cfblk377/1 -> cyemi_362/1
  cyemi_372/1 -> cfblk296/1(cfblk1)
  cfblk349/1 -> cyemi_372/1
  cyemi_373/1 -> cfblk296/2(cfblk11)
  cfblk294/1(cfblk2) -> cyemi_373/1
  cyemi_447/1 -> cfblk297/1(cfblk1)
  cfblk39/1 -> cyemi_447/1
  cyemi_448/1 -> cfblk297/2(cfblk4)
  cfblk370/1 -> cyemi_448/1
  cyemi_450/1 -> cfblk298/1(cfblk1)
  cfblk374/1 -> cyemi_450/1
  cyemi_451/1 -> cfblk298/2(cfblk8)
  cfblk379/1 -> cyemi_451/1
  cyemi_457/1 -> cfblk299/1(cfblk1)
  cyemi_458/1 -> cfblk299/2(cfblk12)
  cfblk369/1 -> cyemi_458/1
  cyemi_459/1 -> cfblk299/3(cfblk13)
  cfblk368/1 -> cyemi_459/1
  cyemi_498/1 -> cfblk3/1
  cfblk236/1 -> cyemi_498/1
  cyemi_499/1 -> cfblk3/2
  cfblk306/2(cfblk12) -> cyemi_499/1
  cyemi_500/1 -> cfblk30/1
  cfblk246/1 -> cyemi_500/1
  cyemi_501/1 -> cfblk300/1(cfblk1)
  cfblk253/1 -> cyemi_501/1
  cyemi_502/1 -> cfblk300/2(cfblk12)
  cfblk19/1 -> cyemi_502/1
  cyemi_517/1 -> cfblk301/1(cfblk1)
  cfblk350/1 -> cyemi_517/1
  cyemi_518/1 -> cfblk301/2(cfblk12)
  cfblk289/1(cfblk2) -> cyemi_518/1
  cyemi_557/1 -> cfblk302/1(cfblk1)
  cfblk113/1 -> cyemi_557/1
  cyemi_595/1 -> cfblk303/1(cfblk1)
  cfblk41/1 -> cyemi_595/1
  cyemi_596/1 -> cfblk303/2(cfblk9)
  cfblk357/1 -> cyemi_596/1
  cyemi_634/1 -> cfblk304/1(cfblk1)
  cfblk371/1 -> cyemi_634/1
  cyemi_635/1 -> cfblk304/2(cfblk7)
  cfblk329/1(cfblk2) -> cyemi_635/1
  cyemi_663/1 -> cfblk305/1(cfblk1)
  cfblk12/1 -> cyemi_663/1
  cyemi_664/1 -> cfblk305/2(cfblk9)
  cfblk361/1 -> cyemi_664/1
  cyemi_665/1 -> cfblk305/3(cfblk10)
  cfblk373/1 -> cyemi_665/1
  cyemi_666/1 -> cfblk305/4(cfblk11)
  cyemi_667/1 -> cfblk305/5(cfblk12)
  cyemi_705/1 -> cfblk306/1(cfblk1)
  cfblk311/2(cfblk12) -> cyemi_705/1
  cyemi_723/1 -> cfblk307/1(cfblk1)
  cfblk93/1 -> cyemi_723/1
  cyemi_724/1 -> cfblk307/2(cfblk12)
  cfblk315/1(cfblk2) -> cyemi_724/1
  cyemi_725/1 -> cfblk307/3(cfblk13)
  cyemi_726/1 -> cfblk307/4(cfblk14)
  cyemi_727/1 -> cfblk307/5(cfblk15)
  cyemi_728/1 -> cfblk307/6(cfblk16)
  cyemi_739/1 -> cfblk308/1(cfblk1)
  cfblk59/1 -> cyemi_739/1
  cyemi_740/1 -> cfblk308/2(cfblk10)
  cyemi_773/1 -> cfblk309/1(cfblk1)
  cfblk344/1(cfblk2) -> cyemi_773/1
  cyemi_774/1 -> cfblk309/2(cfblk13)
  cfblk90/1 -> cyemi_774/1
  cyemi_789/1 -> cfblk31/1
  cfblk32/1 -> cyemi_789/1
  cyemi_790/1 -> cfblk310/1(cfblk1)
  cfblk299/2(cfblk14) -> cyemi_790/1
  cyemi_791/1 -> cfblk310/2(cfblk13)
  cfblk320/2(cfblk13) -> cyemi_791/1
  cyemi_805/1 -> cfblk311/1(cfblk1)
  cfblk300/2(cfblk13) -> cyemi_805/1
  cyemi_806/1 -> cfblk311/2(cfblk9)
  cfblk364/1 -> cyemi_806/1
  cyemi_807/1 -> cfblk311/3(cfblk10)
  cfblk347/1 -> cyemi_807/1
  cyemi_808/1 -> cfblk311/4(cfblk11)
  cfblk250/1 -> cyemi_808/1
  cyemi_816/1 -> cfblk312/1(cfblk1)
  cfblk354/1 -> cyemi_816/1
  cyemi_817/1 -> cfblk312/2(cfblk10)
  cfblk380/1 -> cyemi_817/1
  cyemi_827/1 -> cfblk313/1(cfblk1)
  cfblk232/1 -> cyemi_827/1
  cyemi_828/1 -> cfblk313/2(cfblk13)
  cfblk375/1 -> cyemi_828/1
  cyemi_889/1 -> cfblk314/1(cfblk1)
  cyemi_929/1 -> cfblk315/1(cfblk1)
  cfblk50/1 -> cyemi_929/1
  cyemi_930/1 -> cfblk315/2(cfblk8)
  cfblk36/1 -> cyemi_930/1
  cyemi_931/1 -> cfblk315/3(cfblk9)
  cfblk376/1 -> cyemi_931/1
  cyemi_932/1 -> cfblk315/4(cfblk10)
  cyemi_955/1 -> cfblk316/1(cfblk1)
  cfblk22/1 -> cyemi_955/1
  cyemi_956/1 -> cfblk316/2(cfblk9)
  cfblk338/1(cfblk2) -> cyemi_956/1
  cyemi_963/1 -> cfblk317/1(cfblk1)
  cyemi_970/1 -> cfblk318/1(cfblk1)
  cfblk215/1 -> cyemi_970/1
  cyemi_971/1 -> cfblk318/2(cfblk11)
  cfblk72/1 -> cyemi_971/1
  cyemi_987/1 -> cfblk319/1(cfblk1)
  cfblk49/1 -> cyemi_987/1
  cyemi_988/1 -> cfblk319/2(cfblk14)
  cfblk383/1 -> cyemi_988/1
  cyemi_1002/1 -> cfblk32/1
  cfblk109/1 -> cyemi_1002/1
  cyemi_1003/1 -> cfblk320/1(cfblk1)
  cfblk30/1 -> cyemi_1003/1
  cyemi_1004/1 -> cfblk320/2(cfblk12)
  cfblk301/5(cfblk16) -> cyemi_1004/1
  cyemi_1061/1 -> cfblk321/1(cfblk1)
  cfblk133/1 -> cyemi_1061/1
  cyemi_1062/1 -> cfblk321/2(cfblk6)
  cfblk351/1 -> cyemi_1062/1
  cyemi_1088/1 -> cfblk322/1(cfblk1)
  cyemi_1089/1 -> cfblk322/2(cfblk11)
  cfblk297/4(cfblk7) -> cyemi_1089/1
  cyemi_1103/1 -> cfblk323/1(cfblk1)
  cfblk331/2(cfblk10) -> cyemi_1103/1
  cyemi_1104/1 -> cfblk323/2(cfblk16)
  cfblk101/1 -> cyemi_1104/1
  cyemi_1155/1 -> cfblk324/1(cfblk1)
  cfblk193/1 -> cyemi_1155/1
  cyemi_1156/1 -> cfblk324/2(cfblk8)
  cfblk212/1 -> cyemi_1156/1
  cyemi_1157/1 -> cfblk324/3(cfblk9)
  cfblk76/1 -> cyemi_1157/1
  cyemi_1230/1 -> cfblk325/1(cfblk1)
  cfblk339/1(cfblk2) -> cyemi_1230/1
  cyemi_1231/1 -> cfblk325/2(cfblk6)
  cfblk355/1 -> cyemi_1231/1
  cyemi_1236/1 -> cfblk326/1(cfblk1)
  cfblk91/1 -> cyemi_1236/1
  cyemi_1237/1 -> cfblk326/2(cfblk6)
  cfblk353/1 -> cyemi_1237/1
  cyemi_1238/1 -> cfblk326/3(cfblk7)
  cfblk338/3(cfblk9) -> cyemi_1238/1
  cyemi_1239/1 -> cfblk326/4(cfblk8)
  cyemi_1240/1 -> cfblk326/5(cfblk9)
  cyemi_1246/1 -> cfblk327/1(cfblk1)
  cfblk129/1 -> cyemi_1246/1
  cyemi_1247/1 -> cfblk327/2(cfblk11)
  cfblk296/4(cfblk14) -> cyemi_1247/1
  cyemi_1282/1 -> cfblk328/1(cfblk1)
  cfblk254/1 -> cyemi_1282/1
  cyemi_1283/1 -> cfblk328/2(cfblk7)
  cfblk360/1 -> cyemi_1283/1
  cyemi_1284/1 -> cfblk328/3(cfblk8)
  cyemi_1291/1 -> cfblk329/1(cfblk1)
  cfblk238/1 -> cyemi_1291/1
  cyemi_1292/1 -> cfblk329/2(cfblk10)
  cfblk320/3(cfblk14) -> cyemi_1292/1
  cyemi_1302/1 -> cfblk33/1
  cfblk285/1(cfblk2) -> cyemi_1302/1
  cyemi_1303/1 -> cfblk330/1(cfblk1)
  cfblk293/1(cfblk2) -> cyemi_1303/1
  cyemi_1376/1 -> cfblk331/1(cfblk1)
  cfblk332/3(cfblk11) -> cyemi_1376/1
  cyemi_1377/1 -> cfblk331/2(cfblk9)
  cfblk292/1(cfblk2) -> cyemi_1377/1
  cyemi_1414/1 -> cfblk332/1(cfblk1)
  cfblk248/1 -> cyemi_1414/1
  cyemi_1415/1 -> cfblk332/2(cfblk9)
  cfblk315/2(cfblk11) -> cyemi_1415/1
  cyemi_1423/1 -> cfblk333/1(cfblk1)
  cfblk196/1 -> cyemi_1423/1
  cyemi_1424/1 -> cfblk333/2(cfblk15)
  cyemi_1448/1 -> cfblk334/1(cfblk1)
  cfblk5/1 -> cyemi_1448/1
  cyemi_1449/1 -> cfblk334/2(cfblk6)
  cfblk372/1 -> cyemi_1449/1
  cyemi_1470/1 -> cfblk335/1(cfblk1)
  cfblk306/1(cfblk2) -> cyemi_1470/1
  cyemi_1538/1 -> cfblk336/1(cfblk1)
  cfblk120/1 -> cyemi_1538/1
  cyemi_1546/1 -> cfblk337/1(cfblk1)
  cyemi_1547/1 -> cfblk337/2(cfblk12)
  cfblk363/1 -> cyemi_1547/1
  cyemi_1548/1 -> cfblk337/3(cfblk13)
  cyemi_1560/1 -> cfblk338/1(cfblk1)
  cfblk296/2(cfblk12) -> cyemi_1560/1
  cyemi_1561/1 -> cfblk338/2(cfblk6)
  cfblk329/3(cfblk12) -> cyemi_1561/1
  cyemi_1562/1 -> cfblk338/3(cfblk7)
  cfblk366/1 -> cyemi_1562/1
  cyemi_1567/1 -> cfblk339/1(cfblk1)
  cfblk321/2(cfblk7) -> cyemi_1567/1
  cyemi_1568/1 -> cfblk339/2(cfblk13)
  cyemi_1604/1 -> cfblk34/1
  cfblk117/1 -> cyemi_1604/1
  cyemi_1605/1 -> cfblk340/1(cfblk1)
  cfblk356/1 -> cyemi_1605/1
  cyemi_1639/1 -> cfblk341/1(cfblk1)
  cfblk88/1 -> cyemi_1639/1
  cyemi_1640/1 -> cfblk341/2(cfblk15)
  cfblk300/4(cfblk15) -> cyemi_1640/1
  cyemi_1641/1 -> cfblk341/3(cfblk16)
  cfblk124/1 -> cyemi_1641/1
  cyemi_1683/1 -> cfblk342/1(cfblk1)
  cfblk63/1 -> cyemi_1683/1
  cyemi_1692/1 -> cfblk343/1(cfblk1)
  cfblk235/1 -> cyemi_1692/1
  cyemi_1708/1 -> cfblk344/1(cfblk1)
  cfblk111/1 -> cyemi_1708/1
  cyemi_1709/1 -> cfblk344/2(cfblk12)
  cfblk17/1 -> cyemi_1709/1
  cyemi_1710/1 -> cfblk344/3(cfblk13)
  cyemi_1747/1 -> cfblk345/1
  cfblk105/1 -> cyemi_1747/1
  cyemi_1748/1 -> cfblk346/1
  cfblk300/1(cfblk2) -> cyemi_1748/1
  cyemi_1749/1 -> cfblk347/1
  cfblk291/3(cfblk9) -> cyemi_1749/1
  cyemi_1750/1 -> cfblk348/1
  cfblk64/1 -> cyemi_1750/1
  cyemi_1751/1 -> cfblk349/1
  cfblk322/1(cfblk2) -> cyemi_1751/1
  cyemi_1752/1 -> cfblk35/1
  cfblk324/1(cfblk2) -> cyemi_1752/1
  cyemi_1753/1 -> cfblk350/1
  cyemi_1754/1 -> cfblk351/1
  cfblk292/2(cfblk16) -> cyemi_1754/1
  cyemi_1755/1 -> cfblk352/1
  cfblk309/2(cfblk14) -> cyemi_1755/1
  cyemi_1756/1 -> cfblk353/1
  cfblk341/1(cfblk2) -> cyemi_1756/1
  cyemi_1757/1 -> cfblk354/1
  cfblk326/1(cfblk2) -> cyemi_1757/1
  cyemi_1758/1 -> cfblk355/1
  cyemi_1759/1 -> cfblk356/1
  cfblk304/2(cfblk8) -> cyemi_1759/1
  cyemi_1760/1 -> cfblk357/1
  cfblk332/1(cfblk2) -> cyemi_1760/1
  cyemi_1761/1 -> cfblk358/1
  cfblk62/1 -> cyemi_1761/1
  cyemi_1762/1 -> cfblk359/1
  cfblk100/1 -> cyemi_1762/1
  cyemi_1763/1 -> cfblk36/1
  cfblk216/1 -> cyemi_1763/1
  cyemi_1764/1 -> cfblk360/1
  cfblk77/1 -> cyemi_1764/1
  cyemi_1765/1 -> cfblk361/1
  cfblk302/3(cfblk14) -> cyemi_1765/1
  cyemi_1766/1 -> cfblk362/1
  cfblk317/1(cfblk2) -> cyemi_1766/1
  cyemi_1767/1 -> cfblk363/1
  cfblk317/2(cfblk7) -> cyemi_1767/1
  cyemi_1768/1 -> cfblk364/1
  cfblk337/1(cfblk2) -> cyemi_1768/1
  cyemi_1769/1 -> cfblk365/1
  cfblk86/1 -> cyemi_1769/1
  cyemi_1770/1 -> cfblk366/1
  cfblk287/3(cfblk14) -> cyemi_1770/1
  cyemi_1771/1 -> cfblk367/1
  cfblk333/2(cfblk16) -> cyemi_1771/1
  cyemi_1772/1 -> cfblk368/1
  cfblk333/3(cfblk17) -> cyemi_1772/1
  cyemi_1773/1 -> cfblk369/1
  cfblk123/1 -> cyemi_1773/1
  cyemi_1774/1 -> cfblk37/1
  cfblk309/1(cfblk2) -> cyemi_1774/1
  cyemi_1775/1 -> cfblk370/1
  cfblk313/2(cfblk14) -> cyemi_1775/1
  cyemi_1776/1 -> cfblk371/1
  cfblk43/1 -> cyemi_1776/1
  cyemi_1777/1 -> cfblk372/1
  cyemi_1778/1 -> cfblk373/1
  cyemi_1779/1 -> cfblk374/1
  cfblk334/2(cfblk7) -> cyemi_1779/1
  cyemi_1780/1 -> cfblk375/1
  cfblk53/1 -> cyemi_1780/1
  cyemi_1781/1 -> cfblk376/1
  cfblk339/3(cfblk15) -> cyemi_1781/1
  cyemi_1782/1 -> cfblk377/1
  cfblk315/3(cfblk12) -> cyemi_1782/1
  cyemi_1783/1 -> cfblk378/1
  cfblk295/1(cfblk2) -> cyemi_1783/1
  cyemi_1784/1 -> cfblk379/1
  cfblk321/3(cfblk8) -> cyemi_1784/1
  cyemi_1785/1 -> cfblk38/1
  cfblk13/1 -> cyemi_1785/1
  cyemi_1786/1 -> cfblk38/2
  cfblk78/1 -> cyemi_1786/1
  cyemi_1787/1 -> cfblk380/1
  cfblk3/1 -> cyemi_1787/1
  cyemi_1788/1 -> cfblk381/1
  cfblk311/3(cfblk13) -> cyemi_1788/1
  cyemi_1789/1 -> cfblk382/1
  cfblk300/5(cfblk16) -> cyemi_1789/1
  cyemi_1790/1 -> cfblk383/1
  cfblk329/2(cfblk11) -> cyemi_1790/1
  cyemi_1791/1 -> cfblk384/1
  cfblk329/4(cfblk13) -> cyemi_1791/1
  cyemi_1792/1 -> cfblk385/1
  cfblk200/1 -> cyemi_1792/1
  cyemi_1793/1 -> cfblk39/1
  cfblk1/1 -> cyemi_1793/1
  cyemi_1794/1 -> cfblk39/2
  cfblk345/1 -> cyemi_1794/1
  cyemi_1795/1 -> cfblk4/1
  cfblk297/3(cfblk6) -> cyemi_1795/1
  cyemi_1796/1 -> cfblk40/1
  cfblk94/1 -> cyemi_1796/1
  cyemi_1797/1 -> cfblk41/1
  cfblk291/2(cfblk8) -> cyemi_1797/1
  cyemi_1798/1 -> cfblk42/1
  cfblk26/1 -> cyemi_1798/1
  cyemi_1799/1 -> cfblk43/1
  cfblk54/1 -> cyemi_1799/1
  cyemi_1800/1 -> cfblk44/1
  cfblk335/1(cfblk2) -> cyemi_1800/1
  cyemi_1801/1 -> cfblk45/1
  cfblk127/1 -> cyemi_1801/1
  cyemi_1802/1 -> cfblk46/1
  cfblk203/1 -> cyemi_1802/1
  cyemi_1803/1 -> cfblk46/2
  cfblk40/1 -> cyemi_1803/1
  cyemi_1804/1 -> cfblk47/1
  cfblk316/2(cfblk10) -> cyemi_1804/1
  cyemi_1805/1 -> cfblk48/1
  cfblk241/1 -> cyemi_1805/1
  cyemi_1806/1 -> cfblk49/1
  cfblk339/2(cfblk14) -> cyemi_1806/1
  cyemi_1807/1 -> cfblk5/1
  cfblk4/1 -> cyemi_1807/1
  cyemi_1808/1 -> cfblk50/1
  cfblk223/1 -> cyemi_1808/1
  cyemi_1809/1 -> cfblk51/1
  cfblk75/1 -> cyemi_1809/1
  cyemi_1810/1 -> cfblk51/2
  cfblk23/1 -> cyemi_1810/1
  cyemi_1811/1 -> cfblk52/1
  cyemi_1812/1 -> cfblk53/1
  cfblk14/1 -> cyemi_1812/1
  cyemi_1813/1 -> cfblk54/1
  cfblk285/2(cfblk12) -> cyemi_1813/1
  cyemi_1814/1 -> cfblk55/1
  cfblk218/1 -> cyemi_1814/1
  cyemi_1815/1 -> cfblk56/1
  cfblk328/1(cfblk2) -> cyemi_1815/1
  cyemi_1816/1 -> cfblk57/1
  cfblk305/2(cfblk13) -> cyemi_1816/1
  cyemi_1817/1 -> cfblk58/1
  cfblk209/1 -> cyemi_1817/1
  cyemi_1818/1 -> cfblk58/2
  cfblk300/3(cfblk14) -> cyemi_1818/1
  cyemi_1819/1 -> cfblk59/1
  cfblk33/1 -> cyemi_1819/1
  cyemi_1820/1 -> cfblk6/1
  cfblk24/1 -> cyemi_1820/1
  cyemi_1821/1 -> cfblk60/1
  cfblk310/1(cfblk2) -> cyemi_1821/1
  cyemi_1822/1 -> cfblk61/1
  cfblk96/1 -> cyemi_1822/1
  cyemi_1823/1 -> cfblk62/1
  cfblk332/2(cfblk10) -> cyemi_1823/1
  cyemi_1824/1 -> cfblk63/1
  cfblk210/1 -> cyemi_1824/1
  cyemi_1825/1 -> cfblk64/1
  cfblk37/1 -> cyemi_1825/1
  cyemi_1826/1 -> cfblk64/2
  cfblk288/1(cfblk2) -> cyemi_1826/1
  cyemi_1827/1 -> cfblk65/1
  cfblk73/1 -> cyemi_1827/1
  cyemi_1828/1 -> cfblk66/1
  cfblk336/1(cfblk2) -> cyemi_1828/1
  cyemi_1829/1 -> cfblk67/1
  cfblk35/1 -> cyemi_1829/1
  cyemi_1830/1 -> cfblk68/1
  cfblk198/1 -> cyemi_1830/1
  cyemi_1831/1 -> cfblk69/1
  cfblk342/2(cfblk10) -> cyemi_1831/1
  cyemi_1832/1 -> cfblk7/1
  cfblk207/1 -> cyemi_1832/1
  cyemi_1833/1 -> cfblk70/1
  cfblk325/1(cfblk2) -> cyemi_1833/1
  cyemi_1834/1 -> cfblk71/1
  cfblk192/1 -> cyemi_1834/1
  cyemi_1835/1 -> cfblk72/1
  cfblk110/1 -> cyemi_1835/1
  cyemi_1836/1 -> cfblk73/1
  cfblk237/1 -> cyemi_1836/1
  cyemi_1837/1 -> cfblk74/1
  cfblk102/1 -> cyemi_1837/1
  cyemi_1838/1 -> cfblk75/1
  cfblk97/1 -> cyemi_1838/1
  cyemi_1839/1 -> cfblk76/1
  cfblk301/3(cfblk14) -> cyemi_1839/1
  cyemi_1840/1 -> cfblk77/1
  cfblk318/1(cfblk2) -> cyemi_1840/1
  cyemi_1841/1 -> cfblk77/2
  cfblk329/5(cfblk14) -> cyemi_1841/1
  cyemi_1842/1 -> cfblk78/1
  cfblk132/1 -> cyemi_1842/1
  cyemi_1843/1 -> cfblk79/1
  cfblk233/1 -> cyemi_1843/1
  cyemi_1844/1 -> cfblk8/1
  cfblk330/1(cfblk2) -> cyemi_1844/1
  cyemi_1845/1 -> cfblk80/1
  cfblk299/1(cfblk2) -> cyemi_1845/1
  cyemi_1846/1 -> cfblk81/1
  cyemi_1847/1 -> cfblk82/1
  cfblk71/1 -> cyemi_1847/1
  cyemi_1848/1 -> cfblk83/1
  cfblk297/1(cfblk2) -> cyemi_1848/1
  cyemi_1849/1 -> cfblk84/1
  cfblk89/1 -> cyemi_1849/1
  cyemi_1850/1 -> cfblk85/1
  cfblk292/3(cfblk17) -> cyemi_1850/1
  cyemi_1851/1 -> cfblk86/1
  cfblk95/1 -> cyemi_1851/1
  cyemi_1852/1 -> cfblk87/1
  cfblk247/1 -> cyemi_1852/1
  cyemi_1853/1 -> cfblk88/1
  cyemi_1854/1 -> cfblk89/1
  cfblk298/1(cfblk2) -> cyemi_1854/1
  cyemi_1855/1 -> cfblk89/2
  cfblk126/1 -> cyemi_1855/1
  cyemi_1856/1 -> cfblk9/1
  cfblk116/1 -> cyemi_1856/1
  cyemi_1857/1 -> cfblk90/1
  cfblk321/1(cfblk2) -> cyemi_1857/1
  cyemi_1858/1 -> cfblk91/1
  cfblk220/1 -> cyemi_1858/1
  cyemi_1859/1 -> cfblk92/1
  cfblk288/2(cfblk8) -> cyemi_1859/1
  cyemi_1860/1 -> cfblk92/2
  cyemi_1861/1 -> cfblk93/1
  cfblk66/1 -> cyemi_1861/1
  cyemi_1862/1 -> cfblk93/2
  cfblk288/3(cfblk9) -> cyemi_1862/1
  cyemi_1863/1 -> cfblk94/1
  cfblk234/1 -> cyemi_1863/1
  cyemi_1864/1 -> cfblk95/1
  cfblk287/2(cfblk13) -> cyemi_1864/1
  cyemi_1865/1 -> cfblk95/2
  cfblk313/1(cfblk2) -> cyemi_1865/1
  cyemi_1866/1 -> cfblk96/1
  cfblk290/2(cfblk11) -> cyemi_1866/1
  cyemi_1867/1 -> cfblk97/1
  cyemi_1868/1 -> cfblk98/1
  cfblk322/2(cfblk12) -> cyemi_1868/1
  cyemi_1869/1 -> cfblk98/2
  cyemi_1870/1 -> cfblk99/1

== system equivalent/cfblk204 ==
  Demux : Demux  Tag=STV Demux  Outputs=1
  FromWs : FromWorkspace  Tag=STV FromWs  VariableName=tuvar  SampleTime=0
      SigBuilderData=|
      | common.afterFinalStr = 'Extrapolate'
      | common.sampleTime = 0
      | dataSet.timeRange = [0 10]
      | dataSet.name = 'Group 1'
      | sbobj.Groups.Name = 'Group 1'
      | sbobj.Groups.Signals.Name = 'Signal 1'
      | sbobj.Groups.Signals.XData = [0 4 4 6 6 10]
      | sbobj.Groups.Signals.YData = [0 0 1 1 0 0]
  Signal 1 : Outport  Tag=STV Outport
  wires:
  Demux/1 -> Signal 1/1
  FromWs/1 -> Demux/1

== system equivalent/cfblk228 ==
  Demux : Demux  Tag=STV Demux  Outputs=1
  FromWs : FromWorkspace  Tag=STV FromWs  VariableName=tuvar  SampleTime=0
      SigBuilderData=|
      | common.afterFinalStr = 'Extrapolate'
      | common.sampleTime = 0
      | dataSet.timeRange = [0 10]
      | dataSet.name = 'Group 1'
      | sbobj.Groups.Name = 'Group 1'
      | sbobj.Groups.Signals.Name = 'Signal 1'
      | sbobj.Groups.Signals.XData = [0 4 4 6 6 10]
      | sbobj.Groups.Signals.YData = [0 0 1 1 0 0]
  Signal 1 : Outport  Tag=STV Outport
  wires:
  Demux/1 -> Signal 1/1
  FromWs/1 -> Demux/1

== system equivalent/cfblk242 ==
  Demux : Demux  Tag=STV Demux  Outputs=1
  FromWs : FromWorkspace  Tag=STV FromWs  VariableName=tuvar  SampleTime=0
      SigBuilderData=|
      | common.afterFinalStr = 'Extrapolate'
      | common.sampleTime = 0
      | dataSet.timeRange = [0 10]
      | dataSet.name = 'Group 1'
      | sbobj.Groups.Name = 'Group 1'
      | sbobj.Groups.Signals.Name = 'Signal 1'
      | sbobj.Groups.Signals.XData = [0 4 4 6 6 10]
      | sbobj.Groups.Signals.YData = [0 0 1 1 0 0]
  Signal 1 : Outport  Tag=STV Outport
  wires:
  Demux/1 -> Signal 1/1
  FromWs/1 -> Demux/1

== system equivalent/cfblk285 ==
  cfblk1 : Inport
  cfblk11 : Inport  Port=2
  Action Port : ActionPort  ActionType=then
  cfblk10 : DiscreteTransferFcn
  cfblk13 : Delay
  cfblk3 : DiscreteZeroPole  Poles=[0 0.5]  Gain=1  SampleTime=-1
  cfblk4 : simulink/Discrete/Tapped Delay  vinit=0.0  samptime=-1  NumDelays=1  DelayOrder=Oldest  includeCurrent=off
  cfblk5 : DiscreteTransferFcn
  cfblk6 : simulink/Continuous/PID Controller (2DOF)  Controller=PID  TimeDomain=Discrete-time  SampleTime=-1  IntegratorMethod=Forward Euler  FilterMethod=Forward Euler  Form=Parallel  UseFilter=on  ControllerParametersSource=internal  P=1  I=1  D=0  N=100  b=1  c=1  InitialConditionSource=internal  InitialConditionForIntegrator=0  InitialConditionForFilter=0  ExternalReset=none  LimitOutput=off  UpperSaturationLimit=inf  LowerSaturationLimit=-inf  LinearizeAsGain=off  AntiWindupMode=none  Kb=1  TrackingMode=off  Kt=1  PParamMin=[]  PParamMax=[]  IParamMin=[]  IParamMax=[]  DParamMin=[]  DParamMax=[]  NParamMin=[]  NParamMax=[]  bParamMin=[]  bParamMax=[]  cParamMin=[]  cParamMax=[]  KbParamMin=[]  KbParamMax=[]  KtParamMin=[]  KtParamMax=[]  POutMin=[]  POutMax=[]  IOutMin=[]  IOutMax=[]  DOutMin=[]  DOutMax=[]  NOutMin=[]  NOutMax=[]  bOutMin=[]  bOutMax=[]  cOutMin=[]  cOutMax=[]  KbOutMin=[]  KbOutMax=[]  KtOutMin=[]  KtOutMax=[]  IntegratorOutMin=[]  IntegratorOutMax=[]  FilterOutMin=[]  FilterOutMax=[]  SumOutMin=[]  SumOutMax=[]  Sum1OutMin=[]  Sum1OutMax=[]  Sum2OutMin=[]  Sum2OutMax=[]  Sum3OutMin=[]  Sum3OutMax=[]  SumI1OutMin=[]  SumI1OutMax=[]  SumI2OutMin=[]  SumI2OutMax=[]  SumI3OutMin=[]  SumI3OutMax=[]  SumDOutMin=[]  SumDOutMax=[]  SaturationOutMin=[]  SaturationOutMax=[]  IntegratorContinuousStateAttributes=''  IntegratorStateMustResolveToSignalObject=off  IntegratorRTWStateStorageClass=Auto  FilterContinuousStateAttributes=''  FilterStateMustResolveToSignalObject=off  FilterRTWStateStorageClass=Auto  DifferentiatorICPrevScaledInput=0  DifferentiatorOutMin=[]  DifferentiatorOutMax=[]  FilterDiffOutCoefMin=[]  FilterDiffOutCoefMax=[]  SumDenOutMin=[]  SumDenOutMax=[]  SumNumOutMin=[]  SumNumOutMax=[]  ReciprocalOutMin=[]  ReciprocalOutMax=[]  DivideOutMin=[]  DivideOutMax=[]  TunerSelectOption=Transfer Function Based (PID Tuner App)
  cfblk7 : DiscreteFilter
  cfblk8 : simulink/Discrete/Transfer Fcn Lead or Lag  PoleZ=0.95  ZeroZ=0.75  ICPrevOutput=0.0  ICPrevInput=0.0  DoSatur=off
      settings: SourceProductName=Simulink  SourceProductBaseCode=SL
  cfblk9 : simulink/Continuous/PID Controller  Controller=PID  TimeDomain=Discrete-time  SampleTime=-1  IntegratorMethod=Forward Euler  FilterMethod=Forward Euler  Form=Parallel  UseFilter=on  ControllerParametersSource=internal  P=1  I=1  D=0  N=100  InitialConditionSource=internal  InitialConditionForIntegrator=0  InitialConditionForFilter=0  ExternalReset=none  LimitOutput=off  UpperSaturationLimit=inf  LowerSaturationLimit=-inf  LinearizeAsGain=off  AntiWindupMode=none  Kb=1  TrackingMode=off  Kt=1  PParamMin=[]  PParamMax=[]  IParamMin=[]  IParamMax=[]  DParamMin=[]  DParamMax=[]  NParamMin=[]  NParamMax=[]  KbParamMin=[]  KbParamMax=[]  KtParamMin=[]  KtParamMax=[]  POutMin=[]  POutMax=[]  IOutMin=[]  IOutMax=[]  DOutMin=[]  DOutMax=[]  NOutMin=[]  NOutMax=[]  KbOutMin=[]  KbOutMax=[]  KtOutMin=[]  KtOutMax=[]  IntegratorOutMin=[]  IntegratorOutMax=[]  FilterOutMin=[]  FilterOutMax=[]  SumOutMin=[]  SumOutMax=[]  SumI1OutMin=[]  SumI1OutMax=[]  SumI2OutMin=[]  SumI2OutMax=[]  SumI3OutMin=[]  SumI3OutMax=[]  SumDOutMin=[]  SumDOutMax=[]  SaturationOutMin=[]  SaturationOutMax=[]  IntegratorContinuousStateAttributes=''  IntegratorStateMustResolveToSignalObject=off  IntegratorRTWStateStorageClass=Auto  FilterContinuousStateAttributes=''  FilterStateMustResolveToSignalObject=off  FilterRTWStateStorageClass=Auto  DifferentiatorICPrevScaledInput=0  DifferentiatorOutMin=[]  DifferentiatorOutMax=[]  FilterDiffOutCoefMin=[]  FilterDiffOutCoefMax=[]  SumDenOutMin=[]  SumDenOutMax=[]  SumNumOutMin=[]  SumNumOutMax=[]  ReciprocalOutMin=[]  ReciprocalOutMax=[]  DivideOutMin=[]  DivideOutMax=[]  TunerSelectOption=Transfer Function Based (PID Tuner App)
  cyemi_{114..123} (10 alike) : DataTypeConversion  OutDataTypeStr=double
  cfblk2 : Outport
  cfblk12 : Outport  Port=2
  wires:
  cfblk3/1 -> cyemi_114/1, cyemi_118/1
  cfblk6/1 -> cfblk12/1
  cfblk11/1 -> cfblk2/1
  cyemi_114/1 -> cfblk10/1
  cyemi_115/1 -> cfblk13/1
  cfblk8/1 -> cyemi_115/1
  cyemi_116/1 -> cfblk3/1
  cfblk13/1 -> cyemi_116/1
  cyemi_117/1 -> cfblk4/1
  cfblk7/1 -> cyemi_117/1
  cyemi_118/1 -> cfblk5/1
  cyemi_119/1 -> cfblk6/1
  cfblk9/1 -> cyemi_119/1
  cyemi_120/1 -> cfblk6/2
  cfblk4/1 -> cyemi_120/1
  cyemi_121/1 -> cfblk7/1
  cfblk5/1 -> cyemi_121/1
  cyemi_122/1 -> cfblk8/1
  cfblk10/1 -> cyemi_122/1
  cyemi_123/1 -> cfblk9/1
  cfblk1/1 -> cyemi_123/1
